simulink model "acc_decision_core"  (R2024b)
settings: Solver=FixedStepDiscrete  StartTime=0.0  StopTime=0.05  FixedStep=0.05  RelTol=1e-3
values from neighbouring files (symbols this model uses):
  command_bp = [0 1 2 3 4 5 6 7]    [decision_lookup_data.mat]    (also in generate_decision_lookup_tables.m = commands)
  control_enabled_table = [1 0 0 0 1 1 1 0 1 1 0 0 ... (32 elements, 4x8)]    [decision_lookup_data.mat]    (also in generate_decision_lookup_tables.m = zeros(num_states, num_commands))
  decision_table = [-1 8 8 8 1 5 5 8 2 6 8 8 ... (32 elements, 4x8)]    [decision_lookup_data.mat]    (also in generate_decision_lookup_tables.m = 8 * ones(num_states, num_commands))
  next_state_table = [0 1 2 3 0 0 0 3 0 0 2 3 ... (32 elements, 4x8)]    [decision_lookup_data.mat]    (also in generate_decision_lookup_tables.m = zeros(num_states, num_commands))
  side_effect_table = [0 0 0 0 0 0 1 0 0 0 0 0 ... (32 elements, 4x8)]    [decision_lookup_data.mat]    (also in generate_decision_lookup_tables.m = zeros(num_states, num_commands))
  state_bp = [0 1 2 3]    [decision_lookup_data.mat]    (also in generate_decision_lookup_tables.m = states)
settings Model: Creator=aiden  LastModifiedBy=aiden

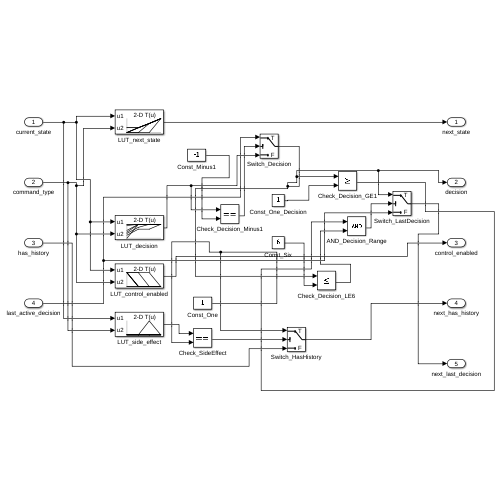
[thumbnail: Simulink's stored preview of the top-level diagram]
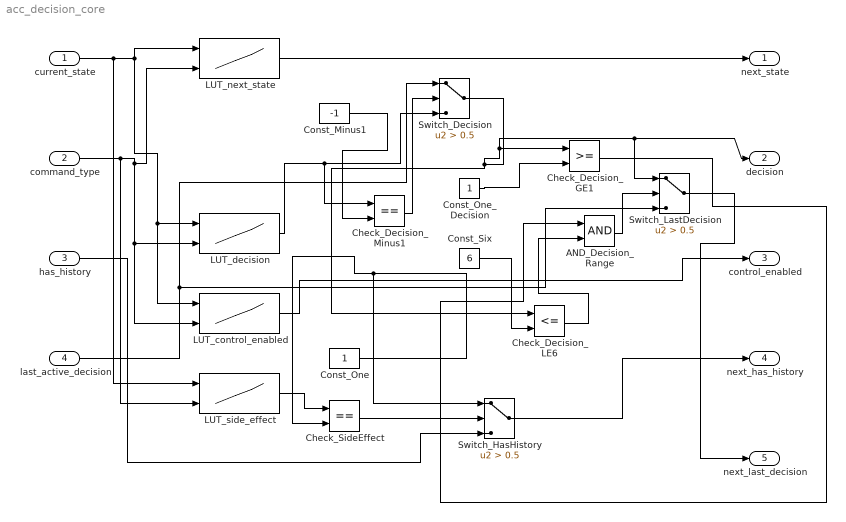
== system acc_decision_core ==
  current_state : Inport
  command_type : Inport  Port=2
  has_history : Inport  Port=3
  last_active_decision : Inport  Port=4
  AND_Decision_Range : Logic  AllPortsSameDT=off  OutDataTypeStr=boolean
  Check_Decision_GE1 : RelationalOperator  OutDataTypeStr=boolean  RndMeth=Simplest  InputSameDT=off
  Check_Decision_LE6 : RelationalOperator  Operator=<=  OutDataTypeStr=boolean  RndMeth=Simplest  InputSameDT=off
  Check_Decision_Minus1 : RelationalOperator  Operator===  OutDataTypeStr=boolean  RndMeth=Simplest  InputSameDT=off
  Check_SideEffect : RelationalOperator  Operator===  OutDataTypeStr=boolean  RndMeth=Simplest  InputSameDT=off
  Const_Minus1 : Constant  Value=-1
  Const_One : Constant
  Const_One_Decision : Constant
  Const_Six : Constant  Value=6
  LUT_control_enabled : Lookup_n-D  BreakpointsForDimension1=state_bp  BreakpointsForDimension2=command_bp  BreakpointsForDimension3=[5, 7]  Table=control_enabled_table  InternalRulePriority=Speed  RndMeth=Simplest
      settings: InputPortMap=u0,u1
  LUT_decision : Lookup_n-D  BreakpointsForDimension1=state_bp  BreakpointsForDimension2=command_bp  BreakpointsForDimension3=[5, 7]  Table=decision_table  InternalRulePriority=Speed  RndMeth=Simplest
      settings: InputPortMap=u0,u1
  LUT_next_state : Lookup_n-D  BreakpointsForDimension1=state_bp  BreakpointsForDimension2=command_bp  BreakpointsForDimension3=[5, 7]  Table=next_state_table  InternalRulePriority=Speed  RndMeth=Simplest
      settings: InputPortMap=u0,u1
  LUT_side_effect : Lookup_n-D  BreakpointsForDimension1=state_bp  BreakpointsForDimension2=command_bp  BreakpointsForDimension3=[5, 7]  Table=side_effect_table  InternalRulePriority=Speed  RndMeth=Simplest
      settings: InputPortMap=u0,u1
  Switch_Decision : Switch  Criteria=u2 > Threshold  Threshold=0.5  SaturateOnIntegerOverflow=off  InputSameDT=off
  Switch_HasHistory : Switch  Criteria=u2 > Threshold  Threshold=0.5  SaturateOnIntegerOverflow=off  InputSameDT=off
  Switch_LastDecision : Switch  Criteria=u2 > Threshold  Threshold=0.5  SaturateOnIntegerOverflow=off  InputSameDT=off
  next_state : Outport
  decision : Outport  Port=2
  control_enabled : Outport  Port=3
  next_has_history : Outport  Port=4
  next_last_decision : Outport  Port=5
  wires:
  current_state/1 -> LUT_decision/1, LUT_control_enabled/1, LUT_next_state/1, LUT_side_effect/1
  command_type/1 -> LUT_decision/2, LUT_control_enabled/2, LUT_next_state/2, LUT_side_effect/2
  LUT_decision/1 -> Check_Decision_Minus1/1, Switch_Decision/3
  Const_Minus1/1 -> Check_Decision_Minus1/2
  Check_Decision_Minus1/1 -> Switch_Decision/2
  last_active_decision/1 -> Switch_Decision/1, Switch_LastDecision/3
  LUT_side_effect/1 -> Check_SideEffect/1
  Const_One/1 -> Check_SideEffect/2, Switch_HasHistory/1
  Check_SideEffect/1 -> Switch_HasHistory/2
  has_history/1 -> Switch_HasHistory/3
  Switch_Decision/1 -> Switch_LastDecision/1, decision/1, Check_Decision_GE1/1, Check_Decision_LE6/1
  Const_One_Decision/1 -> Check_Decision_GE1/2
  Const_Six/1 -> Check_Decision_LE6/2
  Check_Decision_GE1/1 -> AND_Decision_Range/1
  Check_Decision_LE6/1 -> AND_Decision_Range/2
  AND_Decision_Range/1 -> Switch_LastDecision/2
  LUT_next_state/1 -> next_state/1
  LUT_control_enabled/1 -> control_enabled/1
  Switch_HasHistory/1 -> next_has_history/1
  Switch_LastDecision/1 -> next_last_decision/1
